simulink model "aa_IOT"  (R2024b)
settings: Solver=VariableStepAuto  StartTime=0.0  StopTime=0.20  RelTol=1e-3
undefined symbols (not defined in the file): Acid, Ion, Lead, Lithium, sigbuilder_block
libraries: spsBreakerLib x120, spsBatteryLib x72, spsSeriesRLCBranchLib x47, spsVoltageMeasurementLib x33, spsIdealSwitchLib x19, spsDiodeLib x10, spsCurrentMeasurementLib x8, spsThyristorLib x6, sldrtlib x4, spsACVoltageSourceLib x3, spsIGBTLib x2, spsPVArrayLib x1
(part 3 of 7)

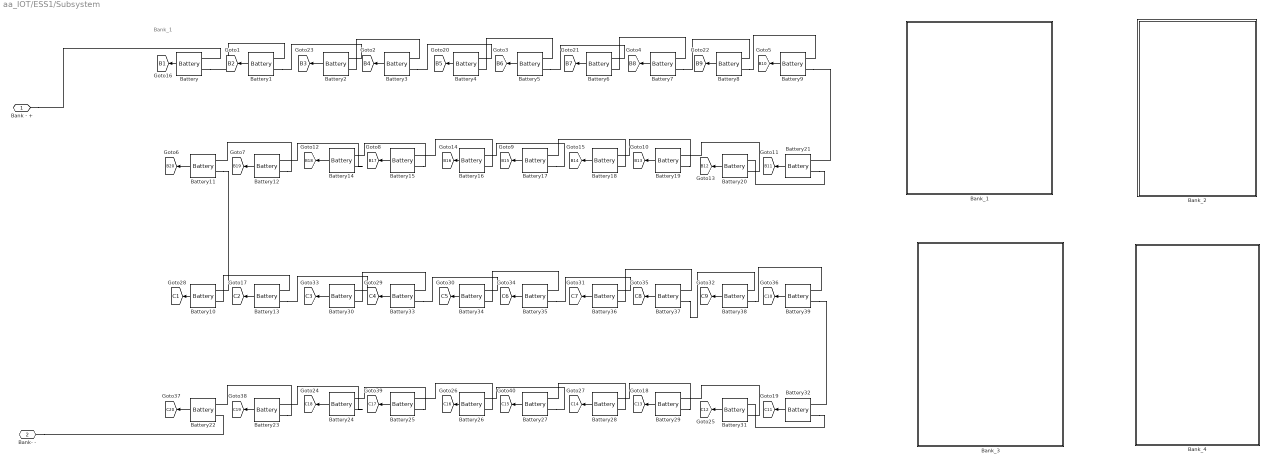
== system aa_IOT/ESS1/Subsystem ==
  note: Bank_1
  Bank_1 : Subsystem
  Bank_2 : Subsystem
  Bank_3 : Subsystem
  Bank_4 : Subsystem
  Battery{,1..39} (40 alike) : spsBatteryLib/Battery  BatType=Lead-Acid  NomV=12  NomQ=100  SOC=80  Batt_Tr=10  PresetModel=on  MaxQ=104.1667  MinV=9  FullV=13.0658  Dis_rate=20  R=0.0012  Normal_OP=31.0278  expZone="[12.2171     0.333333]"
  Bank - + : PMIOPort  Side=Left
  Bank- - : PMIOPort  Port=2  Side=Left
  tag scope: B10=global, B11=global, B12=global, B13=global, B14=global, B15=global, B16=global, B17=global, B18=global, B19=global, B1=global, B20=global, B2=global, B3=global, B4=global, B5=global, B6=global, B7=global, B8=global, B9=global, C10=global, C11=global, C12=global, C13=global, C14=global, C15=global, C16=global, C17=global, C18=global, C19=global, C1=global, C20=global, C2=global, C3=global, C4=global, C5=global, C6=global, C7=global, C8=global, C9=global
  wires:
  Battery1/1 -> [B2]
  Battery5/1 -> [B6]
  Battery25/1 -> [C17]
  Battery20/1 -> [B12]
  Battery34/1 -> [C5]
  Battery28/1 -> [C14]
  Battery4/1 -> [B5]
  Battery16/1 -> [B16]
  Battery2/1 -> [B3]
  Battery18/1 -> [B14]
  Battery14/1 -> [B18]
  Battery8/1 -> [B9]
  Battery6/1 -> [B7]
  Battery17/1 -> [B15]
  Battery24/1 -> [C18]
  Battery9/1 -> [B10]
  Battery12/1 -> [B19]
  Battery15/1 -> [B17]
  Battery21/1 -> [B11]
  Battery11/1 -> [B20]
  Battery10/1 -> [C1]
  Battery19/1 -> [B13]
  Battery3/1 -> [B4]
  Battery7/1 -> [B8]
  Battery27/1 -> [C15]
  Battery13/1 -> [C2]
  Battery/1 -> [B1]
  Battery38/1 -> [C9]
  Battery22/1 -> [C20]
  Battery39/1 -> [C10]
  Battery32/1 -> [C11]
  Battery37/1 -> [C8]
  Battery33/1 -> [C4]
  Battery35/1 -> [C6]
  Battery23/1 -> [C19]
  Battery29/1 -> [C13]
  Battery31/1 -> [C12]
  Battery36/1 -> [C7]
  Battery30/1 -> [C3]
  Battery26/1 -> [C16]
  connections:
  Battery7/LConn2 -- Battery8/LConn1
  Battery20/LConn2 -- Battery19/LConn1
  Battery9/LConn2 -- Battery21/LConn1
  Battery2/LConn2 -- Battery3/LConn1
  Battery13/LConn2 -- Battery30/LConn1
  Battery39/LConn2 -- Battery32/LConn1
  Battery15/LConn2 -- Battery14/LConn1
  Battery16/LConn2 -- Battery15/LConn1
  Battery14/LConn2 -- Battery12/LConn1
  Battery21/LConn2 -- Battery20/LConn1
  Battery6/LConn2 -- Battery7/LConn1
  Battery12/LConn2 -- Battery11/LConn1
  Battery18/LConn2 -- Battery17/LConn1
  Battery17/LConn2 -- Battery16/LConn1
  Battery3/LConn2 -- Battery4/LConn1
  Battery19/LConn2 -- Battery18/LConn1
  Battery8/LConn2 -- Battery9/LConn1
  Battery26/LConn2 -- Battery25/LConn1
  Battery1/LConn2 -- Battery2/LConn1
  Battery4/LConn2 -- Battery5/LConn1
  Battery5/LConn2 -- Battery6/LConn1
  Battery/LConn2 -- Battery1/LConn1
  Battery23/LConn2 -- Battery22/LConn1
  Battery25/LConn2 -- Battery24/LConn1
  Battery10/LConn2 -- Battery13/LConn1
  Battery28/LConn2 -- Battery27/LConn1
  Battery29/LConn2 -- Battery28/LConn1
  Battery33/LConn2 -- Battery34/LConn1
  Battery32/LConn2 -- Battery31/LConn1
  Battery30/LConn2 -- Battery33/LConn1
  Battery34/LConn2 -- Battery35/LConn1
  Battery38/LConn2 -- Battery39/LConn1
  Battery35/LConn2 -- Battery36/LConn1
  Battery24/LConn2 -- Battery23/LConn1
  Battery31/LConn2 -- Battery29/LConn1
  Battery36/LConn2 -- Battery37/LConn1
  Battery37/LConn2 -- Battery38/LConn1
  Battery27/LConn2 -- Battery26/LConn1
  Bank - +/RConn1 -- Battery/LConn1
  Bank- -/RConn1 -- Battery22/LConn2
  Battery11/LConn2 -- Battery10/LConn1

== system aa_IOT/Fast charging controller/Fast charging Switching controller ==
  g1 : Subsystem
  g2 : Subsystem
  g3 : Subsystem
  g4 : Subsystem

== system aa_IOT/Solar/Irradiance  ==
  Demux : Demux  Tag=STV Demux  Outputs=2
      settings: DisplayOption=none
  FromWs : FromWorkspace  Tag=STV FromWs  VariableName=tuvar
      SigBuilderData=|
      | common.afterFinalStr = 'Extrapolate'
      | common.sampleTime = '0'
      | dataSet(1).timeRange = [0 2]
      | dataSet(1).name = 'Constant Irradiance'
      | dataSet(2).timeRange = [0 2]
      | dataSet(2).name = 'Step Irradiance'
      | dataSet(3).timeRange = [0 1]
      | dataSet(3).name = 'Ramp-up/down Irradiance'
      | sbobj.Groups(1).Name = 'Constant Irradiance'
      | sbobj.Groups(1).Signals(1).Name = 'Ir'
      | sbobj.Groups(1).Signals(1).XData = [0 2]
      | sbobj.Groups(1).Signals(1).YData = [1000 1000]
      | sbobj.Groups(1).Signals(2).Name = 'Temp'
      | sbobj.Groups(1).Signals(2).XData = [0 1 1 2]
      | sbobj.Groups(1).Signals(2).YData = [0 0 1 1]
      | sbobj.Groups(1).TimeRange = [0 2]
      | sbobj.Groups(2).Name = 'Step Irradiance'
      | sbobj.Groups(2).Signals(1).Name = 'Ir'
      | sbobj.Groups(2).Signals(1).XData = [0 0.252 0.252 2]
      | sbobj.Groups(2).Signals(1).YData = [600 600 1000 1000]
      | sbobj.Groups(2).Signals(2).Name = 'Temp'
      | sbobj.Groups(2).Signals(2).XData = [0 1 1 2]
      | sbobj.Groups(2).Signals(2).YData = [0 0 1 1]
      | sbobj.Groups(2).TimeRange = [0 2]
      | sbobj.Groups(3).Name = 'Ramp-up/down Irradiance'
      | sbobj.Groups(3).Signals(1).Name = 'Ir'
      | sbobj.Groups(3).Signals(1).XData = [0 0.3 0.3 0.4 0.4 0.5 0.5 1]
      | sbobj.Groups(3).Signals(1).YData = [1000 1000 800 795 600 600 400 395]
      | sbobj.Groups(3).Signals(2).Name = 'Temp'
      | sbobj.Groups(3).Signals(2).XData = [0 1]
      | sbobj.Groups(3).Signals(2).YData = [25 25]
      | sbobj.Groups(3).TimeRange = [0 1]
  Ir : Outport  Tag=STV Outport
  Temp : Outport  Tag=STV Outport  Port=2
  wires:
  Demux/1 -> Ir/1
  FromWs/1 -> Demux/1
  Demux/2 -> Temp/1

== system aa_IOT/Solar/MPPT ==
  "V _ PV " : Inport
  I_PV : Inport  Port=2
  clock : Inport  Port=3
  Embedded MATLAB Function1 : MATLAB Function  TreatAsAtomicUnit=on
  Duty : Outport  VectorParamsAs1DForOutWhenUnconnected=off
  wires:
  Embedded MATLAB Function1/1(D) -> Duty/1
  clock/1 -> Embedded MATLAB Function1/3(T)
  "V _ PV "/1 -> Embedded MATLAB Function1/1(V)
  I_PV/1 -> Embedded MATLAB Function1/2(I)

== system aa_IOT/Solar/Subsystem ==
  Constant : Constant  Value=10000
  Display{1,3..9} (8 alike) : Display
  Mux : Mux  Inputs=8
  Product : Product
  ThingSpeak Output : sldrtlib/Internet of Things/ThingSpeak Output  DrvAddress=2749650  DrvOptions=[1 15 50 66 71 85 71 49 57 55 71 78 77 74 88 48 87 70 97 112 105 46 116 104 105 110 103 115 112 101 97 107 46 99 111 109 0 0 0 0 0 0 0 0 0 0 0 0 0 0 0 0 0 0 0 0 0 0 0 0 0 0 0 0 0 0 0 0 0 0 0 0 0 0 0 0 0 0 0 0 0 0 0 0 0 0 0 0 0 0 0 0 0 0 0 0 0 0 0 0 0 0 0 0 0 0 0 0 0 0 0 0 0 0 0 0 0 0 0 0 0 0 0 0 0 0 0 0 0 0 0 0 0 0 0 0 0 0 0 0 0 0 0 0 0 0 0 0 0 0 0 0 0 0 0 0 0 0 0 0 0 0 0 0 0 0 0 0 0 0 0 0 0 0 0 0 0 0 0 0 0 0 0 0 0 0 0 0 0 0 0 0 0 0 0 0 0 0 0 0 0 0 0 0 0 0 0 0 0 0 0 0 0 0 0 0 0 0 0 0 0 0 0 0 0 0 0 0 0 0 0 0 0 0 0 0 0 0 0 0 0 0 0 0 0 0 0 0 0 0 0 0 0 0 0 0]  SampleTime=0.1  MaxMissedTicks=10000000000000000000000000000000000000000000  ShowMissedTicks=off  YieldWhenWaiting=off  ChannelFields=[1 2 3 4 5 6 7 8]  OptParam=0  InitialValue=[]  FinalValue=[]
  wires:
  [solar_v] -> Mux/1, Display9/1
  [solar_i] -> Mux/2, Display3/1
  [solar_out_p] -> Mux/8, Display7/1
  [solar_irr] -> Mux/5, Display4/1
  [solar_out_i] -> Mux/7, Display8/1
  [solar_out_v] -> Mux/6, Display6/1
  [solar_temp] -> Mux/4, Display5/1
  Mux/1 -> ThingSpeak Output/1
  Product/1 -> Mux/3, Display1/1
  [solar_p] -> Product/2
  Constant/1 -> Product/1

== system aa_IOT/Subsystem/Car Charging Calculator ==
  note: Car Charging Calculator
  note: Car Batttery KWh
  note: Volatge
  note: Current
  note: Time Required in hr
  note: Power in Kw
  note: Power Valiabililty
  Car Battery KWh : Constant  Value=600
  Current : Constant  Value=20
  Display : CustomWebBlock  LabelPosition=Hide  ShowInitialText=on  Configuration="{\"components\":[{\"name\":\"DisplayComponent\",\"settings\":{\"bold\":false,\"font\":\"DSEG7 Classic\",\"fontColor\":[255,255,200],\"fontSize\":\"14\",\"format\":\"short\",\"formatString\":\"%d\",\"italic\":false,\"position\":[0,0,1,1],\"underline\":false}},{\"name\":\"BackgroundImageComponent\",\"settings\":{\"image\":{\"size\":[300,80],\"src\":\"data:image\\/svg+xml;base64,PHN2ZyBpZD0iZnJhbWUiIHhtbG5zPSJodHRwOi8vd3d3LnczLm9yZy8yMDAwL3N2ZyIgeG1sbnM6eGxpbms9Imh0dHA6Ly93d3cudzMub3JnLzE5OTkveGxpbmsiIHZpZXdCb3g9IjAgMCAzODAgMTAxIj48ZGVmcz48c3R5bGU+LmNscy0xe2ZpbGw6IzAwMmI0Mjt9LmNscy0ye2ZpbGw6IzQyNzA4Mjt9LmNscy0ze2ZpbGw6dXJsKCNyYWRpYWwtZ3JhZGllbnQpO308L3N0eWxlPjxyYWRpYWxHcmFkaWVudCBpZD0icmFkaWFsLWdyYWRpZW50IiBjeD0iMTkwIiBjeT0iNTAuNSIgcj0iMjY5LjIxIiBncmFkaWVudFVuaXRzPSJ1c2VyU3BhY2VPblVzZSI+PHN0b3Agb2Zmc2V0PSIwLjAxIiBzdG9wLWNvbG9yPSIjM2U0ZjU4Ii8+PHN0b3Agb2Zmc2V0PSIwLjA2IiBzdG9wLWNvbG9yPSIjNDQ1NzYxIi8+PHN0b3Agb2Zmc2V0PSIwLjE1IiBzdG9wLWNvbG9yPSIjNTU2YTc2Ii8+PHN0b3Agb2Zmc2V0PSIwLjI1IiBzdG9wLWNvbG9yPSIjNmQ4ODk1Ii8+PHN0b3Agb2Zmc2V0PSIwLjM4IiBzdG9wLWNvbG9yPSIjOGZiMmMzIi8+PHN0b3Agb2Zmc2V0PSIwLjUyIiBzdG9wLWNvbG9yPSIjYjZlNGZhIi8+PHN0b3Agb2Zmc2V0PSIxIiBzdG9wLWNvbG9yPSIjMTU0NjU3Ii8+PC9yYWRpYWxHcmFkaWVudD48L2RlZnM+PGcgaWQ9IkxheWVyXzIiIGRhdGEtbmFtZT0iTGF5ZXIgMiI+PGcgaWQ9IkxheWVyXzEtMiIgZGF0YS1uYW1lPSJMYXllciAxLTIiPjxyZWN0IGlkPSJyZWN0MTAzNiIgY2xhc3M9ImNscy0xIiB4PSIxMSIgeT0iMTEiIHdpZHRoPSIzNTgiIGhlaWdodD0iNzkiLz48cGF0aCBpZD0icGF0aDEwMzgiIGNsYXNzPSJjbHMtMiIgZD0iTTgsOFY5M0gzNzJWOFpNMzY5LDkwSDExVjExSDM2OVoiLz48cGF0aCBpZD0icGF0aDEwNDAiIGNsYXNzPSJjbHMtMyIgZD0iTTAsMFYxMDFIMzgwVjBaTTM3Miw5M0g4VjhIMzcyWiIvPjwvZz48L2c+PC9zdmc+\",\"srcOrientation\":\"Right\"},\"position\":[0,0,1,1],\"scaleMode\":\"0\"}},{\"name\":\"ForegroundImageComponent\",\"settings\":{\"angle\":0,\"image\":{\"size\":[0,0],\"src\":\"default\"},\"isForeground\":1,\"position\":[0,0,1,1],\"scaleMode\":\"0\"}}],\"settings\":{\"BindingType\":\"signal\",\"aspectRatio\":1.032258064516129,\"backgroundColor\":[0,0,0,\"1\"],\"backgroundOffset\":0.14,\"backgroundOpacity\":1,\"fixedAspectRatio\":\"on\",\"showBackgroundColor\":false,\"value\":0,\"version\":\"R2023b\"},\"type\":\"Display\"}"
  Display1 : CustomWebBlock  LabelPosition=Hide  ShowInitialText=on  Configuration="{\"components\":[{\"name\":\"DisplayComponent\",\"settings\":{\"bold\":false,\"font\":\"DSEG7 Classic\",\"fontColor\":[255,255,200],\"fontSize\":\"14\",\"format\":\"short\",\"formatString\":\"%d\",\"italic\":false,\"position\":[0,0,1,1],\"underline\":false}},{\"name\":\"BackgroundImageComponent\",\"settings\":{\"image\":{\"size\":[300,80],\"src\":\"data:image\\/svg+xml;base64,PHN2ZyBpZD0iZnJhbWUiIHhtbG5zPSJodHRwOi8vd3d3LnczLm9yZy8yMDAwL3N2ZyIgeG1sbnM6eGxpbms9Imh0dHA6Ly93d3cudzMub3JnLzE5OTkveGxpbmsiIHZpZXdCb3g9IjAgMCAzODAgMTAxIj48ZGVmcz48c3R5bGU+LmNscy0xe2ZpbGw6IzAwMmI0Mjt9LmNscy0ye2ZpbGw6IzQyNzA4Mjt9LmNscy0ze2ZpbGw6dXJsKCNyYWRpYWwtZ3JhZGllbnQpO308L3N0eWxlPjxyYWRpYWxHcmFkaWVudCBpZD0icmFkaWFsLWdyYWRpZW50IiBjeD0iMTkwIiBjeT0iNTAuNSIgcj0iMjY5LjIxIiBncmFkaWVudFVuaXRzPSJ1c2VyU3BhY2VPblVzZSI+PHN0b3Agb2Zmc2V0PSIwLjAxIiBzdG9wLWNvbG9yPSIjM2U0ZjU4Ii8+PHN0b3Agb2Zmc2V0PSIwLjA2IiBzdG9wLWNvbG9yPSIjNDQ1NzYxIi8+PHN0b3Agb2Zmc2V0PSIwLjE1IiBzdG9wLWNvbG9yPSIjNTU2YTc2Ii8+PHN0b3Agb2Zmc2V0PSIwLjI1IiBzdG9wLWNvbG9yPSIjNmQ4ODk1Ii8+PHN0b3Agb2Zmc2V0PSIwLjM4IiBzdG9wLWNvbG9yPSIjOGZiMmMzIi8+PHN0b3Agb2Zmc2V0PSIwLjUyIiBzdG9wLWNvbG9yPSIjYjZlNGZhIi8+PHN0b3Agb2Zmc2V0PSIxIiBzdG9wLWNvbG9yPSIjMTU0NjU3Ii8+PC9yYWRpYWxHcmFkaWVudD48L2RlZnM+PGcgaWQ9IkxheWVyXzIiIGRhdGEtbmFtZT0iTGF5ZXIgMiI+PGcgaWQ9IkxheWVyXzEtMiIgZGF0YS1uYW1lPSJMYXllciAxLTIiPjxyZWN0IGlkPSJyZWN0MTAzNiIgY2xhc3M9ImNscy0xIiB4PSIxMSIgeT0iMTEiIHdpZHRoPSIzNTgiIGhlaWdodD0iNzkiLz48cGF0aCBpZD0icGF0aDEwMzgiIGNsYXNzPSJjbHMtMiIgZD0iTTgsOFY5M0gzNzJWOFpNMzY5LDkwSDExVjExSDM2OVoiLz48cGF0aCBpZD0icGF0aDEwNDAiIGNsYXNzPSJjbHMtMyIgZD0iTTAsMFYxMDFIMzgwVjBaTTM3Miw5M0g4VjhIMzcyWiIvPjwvZz48L2c+PC9zdmc+\",\"srcOrientation\":\"Right\"},\"position\":[0,0,1,1],\"scaleMode\":\"0\"}},{\"name\":\"ForegroundImageComponent\",\"settings\":{\"angle\":0,\"image\":{\"size\":[0,0],\"src\":\"default\"},\"isForeground\":1,\"position\":[0,0,1,1],\"scaleMode\":\"0\"}}],\"settings\":{\"BindingType\":\"signal\",\"aspectRatio\":1.032258064516129,\"backgroundColor\":[0,0,0,\"1\"],\"backgroundOffset\":0.14,\"backgroundOpacity\":1,\"fixedAspectRatio\":\"on\",\"showBackgroundColor\":false,\"value\":0,\"version\":\"R2023b\"},\"type\":\"Display\"}"
  Display2 : CustomWebBlock  LabelPosition=Hide  ShowInitialText=on  Configuration="{\"components\":[{\"name\":\"DisplayComponent\",\"settings\":{\"bold\":false,\"font\":\"DSEG7 Classic\",\"fontColor\":[255,255,200],\"fontSize\":\"14\",\"format\":\"short\",\"formatString\":\"%d\",\"italic\":false,\"position\":[0,0,1,1],\"underline\":false}},{\"name\":\"BackgroundImageComponent\",\"settings\":{\"image\":{\"size\":[300,80],\"src\":\"data:image\\/svg+xml;base64,PHN2ZyBpZD0iZnJhbWUiIHhtbG5zPSJodHRwOi8vd3d3LnczLm9yZy8yMDAwL3N2ZyIgeG1sbnM6eGxpbms9Imh0dHA6Ly93d3cudzMub3JnLzE5OTkveGxpbmsiIHZpZXdCb3g9IjAgMCAzODAgMTAxIj48ZGVmcz48c3R5bGU+LmNscy0xe2ZpbGw6IzAwMmI0Mjt9LmNscy0ye2ZpbGw6IzQyNzA4Mjt9LmNscy0ze2ZpbGw6dXJsKCNyYWRpYWwtZ3JhZGllbnQpO308L3N0eWxlPjxyYWRpYWxHcmFkaWVudCBpZD0icmFkaWFsLWdyYWRpZW50IiBjeD0iMTkwIiBjeT0iNTAuNSIgcj0iMjY5LjIxIiBncmFkaWVudFVuaXRzPSJ1c2VyU3BhY2VPblVzZSI+PHN0b3Agb2Zmc2V0PSIwLjAxIiBzdG9wLWNvbG9yPSIjM2U0ZjU4Ii8+PHN0b3Agb2Zmc2V0PSIwLjA2IiBzdG9wLWNvbG9yPSIjNDQ1NzYxIi8+PHN0b3Agb2Zmc2V0PSIwLjE1IiBzdG9wLWNvbG9yPSIjNTU2YTc2Ii8+PHN0b3Agb2Zmc2V0PSIwLjI1IiBzdG9wLWNvbG9yPSIjNmQ4ODk1Ii8+PHN0b3Agb2Zmc2V0PSIwLjM4IiBzdG9wLWNvbG9yPSIjOGZiMmMzIi8+PHN0b3Agb2Zmc2V0PSIwLjUyIiBzdG9wLWNvbG9yPSIjYjZlNGZhIi8+PHN0b3Agb2Zmc2V0PSIxIiBzdG9wLWNvbG9yPSIjMTU0NjU3Ii8+PC9yYWRpYWxHcmFkaWVudD48L2RlZnM+PGcgaWQ9IkxheWVyXzIiIGRhdGEtbmFtZT0iTGF5ZXIgMiI+PGcgaWQ9IkxheWVyXzEtMiIgZGF0YS1uYW1lPSJMYXllciAxLTIiPjxyZWN0IGlkPSJyZWN0MTAzNiIgY2xhc3M9ImNscy0xIiB4PSIxMSIgeT0iMTEiIHdpZHRoPSIzNTgiIGhlaWdodD0iNzkiLz48cGF0aCBpZD0icGF0aDEwMzgiIGNsYXNzPSJjbHMtMiIgZD0iTTgsOFY5M0gzNzJWOFpNMzY5LDkwSDExVjExSDM2OVoiLz48cGF0aCBpZD0icGF0aDEwNDAiIGNsYXNzPSJjbHMtMyIgZD0iTTAsMFYxMDFIMzgwVjBaTTM3Miw5M0g4VjhIMzcyWiIvPjwvZz48L2c+PC9zdmc+\",\"srcOrientation\":\"Right\"},\"position\":[0,0,1,1],\"scaleMode\":\"0\"}},{\"name\":\"ForegroundImageComponent\",\"settings\":{\"angle\":0,\"image\":{\"size\":[0,0],\"src\":\"default\"},\"isForeground\":1,\"position\":[0,0,1,1],\"scaleMode\":\"0\"}}],\"settings\":{\"BindingType\":\"signal\",\"aspectRatio\":1.032258064516129,\"backgroundColor\":[0,0,0,\"1\"],\"backgroundOffset\":0.14,\"backgroundOpacity\":1,\"fixedAspectRatio\":\"on\",\"showBackgroundColor\":false,\"value\":0,\"version\":\"R2023b\"},\"type\":\"Display\"}"
  Display3 : CustomWebBlock  LabelPosition=Hide  ShowInitialText=on  Configuration="{\"components\":[{\"name\":\"DisplayComponent\",\"settings\":{\"bold\":false,\"font\":\"DSEG7 Classic\",\"fontColor\":[255,255,200],\"fontSize\":\"14\",\"format\":\"shortG\",\"formatString\":\"%d\",\"italic\":false,\"position\":[0,0,1,1],\"underline\":false}},{\"name\":\"BackgroundImageComponent\",\"settings\":{\"image\":{\"size\":[300,80],\"src\":\"data:image\\/svg+xml;base64,PHN2ZyBpZD0iZnJhbWUiIHhtbG5zPSJodHRwOi8vd3d3LnczLm9yZy8yMDAwL3N2ZyIgeG1sbnM6eGxpbms9Imh0dHA6Ly93d3cudzMub3JnLzE5OTkveGxpbmsiIHZpZXdCb3g9IjAgMCAzODAgMTAxIj48ZGVmcz48c3R5bGU+LmNscy0xe2ZpbGw6IzAwMmI0Mjt9LmNscy0ye2ZpbGw6IzQyNzA4Mjt9LmNscy0ze2ZpbGw6dXJsKCNyYWRpYWwtZ3JhZGllbnQpO308L3N0eWxlPjxyYWRpYWxHcmFkaWVudCBpZD0icmFkaWFsLWdyYWRpZW50IiBjeD0iMTkwIiBjeT0iNTAuNSIgcj0iMjY5LjIxIiBncmFkaWVudFVuaXRzPSJ1c2VyU3BhY2VPblVzZSI+PHN0b3Agb2Zmc2V0PSIwLjAxIiBzdG9wLWNvbG9yPSIjM2U0ZjU4Ii8+PHN0b3Agb2Zmc2V0PSIwLjA2IiBzdG9wLWNvbG9yPSIjNDQ1NzYxIi8+PHN0b3Agb2Zmc2V0PSIwLjE1IiBzdG9wLWNvbG9yPSIjNTU2YTc2Ii8+PHN0b3Agb2Zmc2V0PSIwLjI1IiBzdG9wLWNvbG9yPSIjNmQ4ODk1Ii8+PHN0b3Agb2Zmc2V0PSIwLjM4IiBzdG9wLWNvbG9yPSIjOGZiMmMzIi8+PHN0b3Agb2Zmc2V0PSIwLjUyIiBzdG9wLWNvbG9yPSIjYjZlNGZhIi8+PHN0b3Agb2Zmc2V0PSIxIiBzdG9wLWNvbG9yPSIjMTU0NjU3Ii8+PC9yYWRpYWxHcmFkaWVudD48L2RlZnM+PGcgaWQ9IkxheWVyXzIiIGRhdGEtbmFtZT0iTGF5ZXIgMiI+PGcgaWQ9IkxheWVyXzEtMiIgZGF0YS1uYW1lPSJMYXllciAxLTIiPjxyZWN0IGlkPSJyZWN0MTAzNiIgY2xhc3M9ImNscy0xIiB4PSIxMSIgeT0iMTEiIHdpZHRoPSIzNTgiIGhlaWdodD0iNzkiLz48cGF0aCBpZD0icGF0aDEwMzgiIGNsYXNzPSJjbHMtMiIgZD0iTTgsOFY5M0gzNzJWOFpNMzY5LDkwSDExVjExSDM2OVoiLz48cGF0aCBpZD0icGF0aDEwNDAiIGNsYXNzPSJjbHMtMyIgZD0iTTAsMFYxMDFIMzgwVjBaTTM3Miw5M0g4VjhIMzcyWiIvPjwvZz48L2c+PC9zdmc+\",\"srcOrientation\":\"Right\"},\"position\":[0,0,1,1],\"scaleMode\":\"0\"}},{\"name\":\"ForegroundImageComponent\",\"settings\":{\"angle\":0,\"image\":{\"size\":[0,0],\"src\":\"default\"},\"isForeground\":1,\"position\":[0,0,1,1],\"scaleMode\":\"0\"}}],\"settings\":{\"BindingType\":\"signal\",\"aspectRatio\":1.032258064516129,\"backgroundColor\":[0,0,0,\"1\"],\"backgroundOffset\":0.14,\"backgroundOpacity\":1,\"fixedAspectRatio\":\"on\",\"showBackgroundColor\":false,\"value\":0,\"version\":\"R2023b\"},\"type\":\"Display\"}"
  Display4 : CustomWebBlock  LabelPosition=Hide  ShowInitialText=on  Configuration="{\"components\":[{\"name\":\"DisplayComponent\",\"settings\":{\"bold\":false,\"font\":\"DSEG7 Classic\",\"fontColor\":[255,255,200],\"fontSize\":\"14\",\"format\":\"shortG\",\"formatString\":\"%d\",\"italic\":false,\"position\":[0,0,1,1],\"underline\":false}},{\"name\":\"BackgroundImageComponent\",\"settings\":{\"image\":{\"size\":[300,80],\"src\":\"data:image\\/svg+xml;base64,PHN2ZyBpZD0iZnJhbWUiIHhtbG5zPSJodHRwOi8vd3d3LnczLm9yZy8yMDAwL3N2ZyIgeG1sbnM6eGxpbms9Imh0dHA6Ly93d3cudzMub3JnLzE5OTkveGxpbmsiIHZpZXdCb3g9IjAgMCAzODAgMTAxIj48ZGVmcz48c3R5bGU+LmNscy0xe2ZpbGw6IzAwMmI0Mjt9LmNscy0ye2ZpbGw6IzQyNzA4Mjt9LmNscy0ze2ZpbGw6dXJsKCNyYWRpYWwtZ3JhZGllbnQpO308L3N0eWxlPjxyYWRpYWxHcmFkaWVudCBpZD0icmFkaWFsLWdyYWRpZW50IiBjeD0iMTkwIiBjeT0iNTAuNSIgcj0iMjY5LjIxIiBncmFkaWVudFVuaXRzPSJ1c2VyU3BhY2VPblVzZSI+PHN0b3Agb2Zmc2V0PSIwLjAxIiBzdG9wLWNvbG9yPSIjM2U0ZjU4Ii8+PHN0b3Agb2Zmc2V0PSIwLjA2IiBzdG9wLWNvbG9yPSIjNDQ1NzYxIi8+PHN0b3Agb2Zmc2V0PSIwLjE1IiBzdG9wLWNvbG9yPSIjNTU2YTc2Ii8+PHN0b3Agb2Zmc2V0PSIwLjI1IiBzdG9wLWNvbG9yPSIjNmQ4ODk1Ii8+PHN0b3Agb2Zmc2V0PSIwLjM4IiBzdG9wLWNvbG9yPSIjOGZiMmMzIi8+PHN0b3Agb2Zmc2V0PSIwLjUyIiBzdG9wLWNvbG9yPSIjYjZlNGZhIi8+PHN0b3Agb2Zmc2V0PSIxIiBzdG9wLWNvbG9yPSIjMTU0NjU3Ii8+PC9yYWRpYWxHcmFkaWVudD48L2RlZnM+PGcgaWQ9IkxheWVyXzIiIGRhdGEtbmFtZT0iTGF5ZXIgMiI+PGcgaWQ9IkxheWVyXzEtMiIgZGF0YS1uYW1lPSJMYXllciAxLTIiPjxyZWN0IGlkPSJyZWN0MTAzNiIgY2xhc3M9ImNscy0xIiB4PSIxMSIgeT0iMTEiIHdpZHRoPSIzNTgiIGhlaWdodD0iNzkiLz48cGF0aCBpZD0icGF0aDEwMzgiIGNsYXNzPSJjbHMtMiIgZD0iTTgsOFY5M0gzNzJWOFpNMzY5LDkwSDExVjExSDM2OVoiLz48cGF0aCBpZD0icGF0aDEwNDAiIGNsYXNzPSJjbHMtMyIgZD0iTTAsMFYxMDFIMzgwVjBaTTM3Miw5M0g4VjhIMzcyWiIvPjwvZz48L2c+PC9zdmc+\",\"srcOrientation\":\"Right\"},\"position\":[0,0,1,1],\"scaleMode\":\"0\"}},{\"name\":\"ForegroundImageComponent\",\"settings\":{\"angle\":0,\"image\":{\"size\":[0,0],\"src\":\"default\"},\"isForeground\":1,\"position\":[0,0,1,1],\"scaleMode\":\"0\"}}],\"settings\":{\"BindingType\":\"signal\",\"aspectRatio\":1.032258064516129,\"backgroundColor\":[0,0,0,\"1\"],\"backgroundOffset\":0.14,\"backgroundOpacity\":1,\"fixedAspectRatio\":\"on\",\"showBackgroundColor\":false,\"value\":0,\"version\":\"R2023b\"},\"type\":\"Display\"}"
  Lamp : LampBlock  Icon=Check2
  Power : Display
  Subsystem9 : Subsystem
  Time : Display
  Voltage : Constant  Value=240
  wires:
  Voltage/1 -> Subsystem9/2(In2)
  Current/1 -> Subsystem9/3(In3)
  Subsystem9/1(Out1) -> Time/1
  Car Battery KWh/1 -> Subsystem9/1(In1)
  Subsystem9/2(Out2) -> Power/1

== system aa_IOT/Subsystem11/. ==
  Battery : spsBatteryLib/Battery  BatType=Lithium-Ion  NomV=12  NomQ=10  SOC=95  Batt_Tr=30  PresetModel=on  MaxQ=10  MinV=9  FullV=13.9678  Dis_rate=4.3478  R=0.012  Normal_OP=9.0435  expZone="[12.9646     0.491304]"
  Breaker{,1..3} (4 alike) : spsBreakerLib/Breaker  InitialState=0  SwitchingTimes="[1/60  5/60]"  External=on  BreakerResistance=0.01  SnubberResistance=1e6  SnubberCapacitance=inf  Measurements=None  MoreParameters=on  NoBreakLoop=off
  Bus Selector : BusSelector  OutputSignals=SOC (%),Current (A),Voltage (V)
  Constant : Constant  Value=1000000
  Constant1 : Constant  Value=30
  Product : Product
  Scope : Scope  NumInputPorts=3
  Series RLC Branch : spsSeriesRLCBranchLib/Series RLC Branch  LConnTagsString=__new0  RConnTagsString=__new0  BranchType=R  Resistance=1  Inductance=1e-3  SetiL0=off  InitialCurrent=0  Capacitance=1e-6  Setx0=off  InitialVoltage=0  Measurements=None
  + : PMIOPort  Side=Right
  - : PMIOPort  Port=2  Side=Right
  tag scope: batt_ava=global, batt_power=global, batt_soc=global, batt_voltage=global, s1=global
  wires:
  Battery/1 -> Bus Selector/1
  [c1] -> Breaker3/1, Breaker/1
  [d1] -> Breaker1/1, Breaker2/1
  Bus Selector/3 -> [batt_voltage], Scope/3  "<Voltage (V)>"
  Bus Selector/1 -> [s1], [batt_soc], Scope/1  "<SOC (%)>"
  Bus Selector/2 -> Product/1  "<Current (A)>"
  Constant/1 -> Product/2
  Product/1 -> [batt_power], Scope/2
  Constant1/1 -> [batt_ava]
  connections:
  Breaker2/LConn1 -- Breaker3/RConn1 -- Battery/LConn2
  Breaker1/LConn1 -- Battery/LConn1 -- Breaker/RConn1
  +/RConn1 -- Breaker/LConn1
  Series RLC Branch/LConn1 -- Breaker2/RConn1
  Series RLC Branch/RConn1 -- Breaker1/RConn1
  -/RConn1 -- Breaker3/LConn1

== system aa_IOT/Subsystem11/DC - DC Converter ==
  C : spsSeriesRLCBranchLib/Series RLC Branch  LConnTagsString=__new0  RConnTagsString=__new0  BranchType=C  Resistance=0.01  Inductance=1e-3  SetiL0=off  InitialCurrent=0  Capacitance=1000e-6  Setx0=on  InitialVoltage=200  Measurements=None
  Diode : spsDiodeLib/Diode  Ron=0.001  Lon=0  Vf=1.1  IC=0  UseSnubber=off  Rs=500  Cs=250e-9  Measurements=off
  Diode2 : spsDiodeLib/Diode  Ron=0.001  Lon=0  Vf=0.7  IC=0  UseSnubber=off  Rs=500  Cs=250e-9  Measurements=off
  Display1 : Display
  Display2 : Display
  IGBT : spsIGBTLib/IGBT  Ron=0.001  Lon=0  Vf=1.1  Tf=1e-6  Tt=2e-6  IC=0  Rs=1e5  Cs=inf  Measurements=off
  Pulse Generator : DiscretePulseGenerator  PulseType=Time based  Period=10  PulseWidth=5
  RL : spsSeriesRLCBranchLib/Series RLC Branch  LConnTagsString=__new0  RConnTagsString=__new0  BranchType=RL  Resistance=0.05  Inductance=470e-6  SetiL0=off  InitialCurrent=0  Capacitance=1e-6  Setx0=off  InitialVoltage=0  Measurements=None
  Voltage Measurement1 : spsVoltageMeasurementLib/Voltage Measurement  PhasorSimulation=off  OutputType=Complex  PSBequivalent=0
  Voltage Measurement2 : spsVoltageMeasurementLib/Voltage Measurement  PhasorSimulation=off  OutputType=Complex  PSBequivalent=0
  DC + : PMIOPort  Side=Right
  solar panel + : PMIOPort  Port=2  Side=Left
  solar panel - : PMIOPort  Port=3  Side=Left
  DC - : PMIOPort  Port=4  Side=Right
  wires:
  Pulse Generator/1 -> IGBT/1
  Voltage Measurement1/1 -> Display1/1
  Voltage Measurement2/1 -> Display2/1
  connections:
  DC +/RConn1 -- Diode/RConn1 -- Voltage Measurement2/LConn1
  Diode2/RConn1 -- C/LConn1 -- RL/LConn1
  Diode/LConn1 -- RL/RConn1 -- IGBT/LConn1
  Diode2/LConn1 -- solar panel +/RConn1 -- Voltage Measurement1/LConn1
  DC -/RConn1 -- C/RConn1 -- Voltage Measurement1/LConn2 -- solar panel -/RConn1 -- IGBT/RConn1 -- Voltage Measurement2/LConn2

== system aa_IOT/Subsystem11/Subsystem ==
  Battery : spsBatteryLib/Battery  BatType=Lithium-Ion  NomV=12  NomQ=10  SOC=95  Batt_Tr=30  PresetModel=on  MaxQ=10  MinV=9  FullV=13.9678  Dis_rate=4.3478  R=0.012  Normal_OP=9.0435  expZone="[12.9646     0.491304]"
  Breaker{,1..3} (4 alike) : spsBreakerLib/Breaker  InitialState=0  SwitchingTimes="[1/60  5/60]"  External=on  BreakerResistance=0.01  SnubberResistance=1e6  SnubberCapacitance=inf  Measurements=None  MoreParameters=on  NoBreakLoop=off
  Bus Selector : BusSelector  OutputSignals=SOC (%),Current (A),Voltage (V)
  Scope : Scope  NumInputPorts=3
  Series RLC Branch : spsSeriesRLCBranchLib/Series RLC Branch  LConnTagsString=__new0  RConnTagsString=__new0  BranchType=R  Resistance=1  Inductance=1e-3  SetiL0=off  InitialCurrent=0  Capacitance=1e-6  Setx0=off  InitialVoltage=0  Measurements=None
  + : PMIOPort  Side=Right
  - : PMIOPort  Port=2  Side=Right
  tag scope: s5=global
  wires:
  Battery/1 -> Bus Selector/1
  [c5] -> Breaker3/1, Breaker/1
  Bus Selector/2 -> Scope/2  "<Current (A)>"
  [d5] -> Breaker1/1, Breaker2/1
  Bus Selector/3 -> Scope/3  "<Voltage (V)>"
  Bus Selector/1 -> [s5], Scope/1  "<SOC (%)>"
  connections:
  Breaker2/LConn1 -- Breaker3/RConn1 -- Battery/LConn2
  Breaker1/LConn1 -- Battery/LConn1 -- Breaker/RConn1
  +/RConn1 -- Breaker/LConn1
  Series RLC Branch/LConn1 -- Breaker2/RConn1
  Series RLC Branch/RConn1 -- Breaker1/RConn1
  -/RConn1 -- Breaker3/LConn1

== system aa_IOT/Subsystem11/Subsystem10 ==
  Battery : spsBatteryLib/Battery  BatType=Lithium-Ion  NomV=12  NomQ=10  SOC=95  Batt_Tr=30  PresetModel=on  MaxQ=10  MinV=9  FullV=13.9678  Dis_rate=4.3478  R=0.012  Normal_OP=9.0435  expZone="[12.9646     0.491304]"
  Breaker{,1..3} (4 alike) : spsBreakerLib/Breaker  InitialState=0  SwitchingTimes="[1/60  5/60]"  External=on  BreakerResistance=0.01  SnubberResistance=1e6  SnubberCapacitance=inf  Measurements=None  MoreParameters=on  NoBreakLoop=off
  Bus Selector : BusSelector  OutputSignals=SOC (%),Current (A),Voltage (V)
  Display : Display
  MATLAB Function : MATLAB Function  TreatAsAtomicUnit=on
  Scope : Scope  NumInputPorts=3
  Series RLC Branch : spsSeriesRLCBranchLib/Series RLC Branch  LConnTagsString=__new0  RConnTagsString=__new0  BranchType=R  Resistance=1  Inductance=1e-3  SetiL0=off  InitialCurrent=0  Capacitance=1e-6  Setx0=off  InitialVoltage=0  Measurements=None
  + : PMIOPort  Side=Right
  - : PMIOPort  Port=2  Side=Right
  tag scope: s16=global
  wires:
  Battery/1 -> Bus Selector/1
  [c16] -> Breaker3/1, Breaker/1
  Bus Selector/2 -> MATLAB Function/3(Current), Scope/2  "<Current (A)>"
  [d16] -> Breaker1/1, Breaker2/1
  Bus Selector/3 -> MATLAB Function/2(Voltage), Scope/3  "<Voltage (V)>"
  Bus Selector/1 -> [s16], MATLAB Function/1(SOC), Scope/1  "<SOC (%)>"
  MATLAB Function/1(output) -> Display/1
  connections:
  Breaker2/LConn1 -- Breaker3/RConn1 -- Battery/LConn2
  Breaker1/LConn1 -- Battery/LConn1 -- Breaker/RConn1
  +/RConn1 -- Breaker/LConn1
  Series RLC Branch/LConn1 -- Breaker2/RConn1
  Series RLC Branch/RConn1 -- Breaker1/RConn1
  -/RConn1 -- Breaker3/LConn1

== system aa_IOT/Subsystem11/Subsystem11 ==
  Battery : spsBatteryLib/Battery  BatType=Lithium-Ion  NomV=12  NomQ=10  SOC=95  Batt_Tr=30  PresetModel=on  MaxQ=10  MinV=9  FullV=13.9678  Dis_rate=4.3478  R=0.012  Normal_OP=9.0435  expZone="[12.9646     0.491304]"
  Breaker{,1..3} (4 alike) : spsBreakerLib/Breaker  InitialState=0  SwitchingTimes="[1/60  5/60]"  External=on  BreakerResistance=0.01  SnubberResistance=1e6  SnubberCapacitance=inf  Measurements=None  MoreParameters=on  NoBreakLoop=off
  Bus Selector : BusSelector  OutputSignals=SOC (%),Current (A),Voltage (V)
  Display : Display
  MATLAB Function : MATLAB Function  TreatAsAtomicUnit=on
  Scope : Scope  NumInputPorts=3
  Series RLC Branch : spsSeriesRLCBranchLib/Series RLC Branch  LConnTagsString=__new0  RConnTagsString=__new0  BranchType=R  Resistance=1  Inductance=1e-3  SetiL0=off  InitialCurrent=0  Capacitance=1e-6  Setx0=off  InitialVoltage=0  Measurements=None
  + : PMIOPort  Side=Right
  - : PMIOPort  Port=2  Side=Right
  tag scope: s18=global
  wires:
  Battery/1 -> Bus Selector/1
  [c18] -> Breaker3/1, Breaker/1
  Bus Selector/2 -> MATLAB Function/3(Current), Scope/2  "<Current (A)>"
  [d18] -> Breaker1/1, Breaker2/1
  Bus Selector/3 -> MATLAB Function/2(Voltage), Scope/3  "<Voltage (V)>"
  Bus Selector/1 -> [s18], MATLAB Function/1(SOC), Scope/1  "<SOC (%)>"
  MATLAB Function/1(output) -> Display/1
  connections:
  Breaker2/LConn1 -- Breaker3/RConn1 -- Battery/LConn2
  Breaker1/LConn1 -- Battery/LConn1 -- Breaker/RConn1
  +/RConn1 -- Breaker/LConn1
  Series RLC Branch/LConn1 -- Breaker2/RConn1
  Series RLC Branch/RConn1 -- Breaker1/RConn1
  -/RConn1 -- Breaker3/LConn1

== system aa_IOT/Subsystem11/Subsystem12 ==
  Battery : spsBatteryLib/Battery  BatType=Lithium-Ion  NomV=12  NomQ=10  SOC=95  Batt_Tr=30  PresetModel=on  MaxQ=10  MinV=9  FullV=13.9678  Dis_rate=4.3478  R=0.012  Normal_OP=9.0435  expZone="[12.9646     0.491304]"
  Breaker{,1..3} (4 alike) : spsBreakerLib/Breaker  InitialState=0  SwitchingTimes="[1/60  5/60]"  External=on  BreakerResistance=0.01  SnubberResistance=1e6  SnubberCapacitance=inf  Measurements=None  MoreParameters=on  NoBreakLoop=off
  Bus Selector : BusSelector  OutputSignals=SOC (%),Current (A),Voltage (V)
  Scope : Scope  NumInputPorts=3
  Series RLC Branch : spsSeriesRLCBranchLib/Series RLC Branch  LConnTagsString=__new0  RConnTagsString=__new0  BranchType=R  Resistance=1  Inductance=1e-3  SetiL0=off  InitialCurrent=0  Capacitance=1e-6  Setx0=off  InitialVoltage=0  Measurements=None
  + : PMIOPort  Side=Right
  - : PMIOPort  Port=2  Side=Right
  tag scope: s17=global
  wires:
  Battery/1 -> Bus Selector/1
  [c17] -> Breaker3/1, Breaker/1
  Bus Selector/2 -> Scope/2  "<Current (A)>"
  [d17] -> Breaker1/1, Breaker2/1
  Bus Selector/3 -> Scope/3  "<Voltage (V)>"
  Bus Selector/1 -> [s17], Scope/1  "<SOC (%)>"
  connections:
  Breaker2/LConn1 -- Breaker3/RConn1 -- Battery/LConn2
  Breaker1/LConn1 -- Battery/LConn1 -- Breaker/RConn1
  +/RConn1 -- Breaker/LConn1
  Series RLC Branch/LConn1 -- Breaker2/RConn1
  Series RLC Branch/RConn1 -- Breaker1/RConn1
  -/RConn1 -- Breaker3/LConn1

== system aa_IOT/Subsystem11/Subsystem13 ==
  Battery : spsBatteryLib/Battery  BatType=Lithium-Ion  NomV=12  NomQ=10  SOC=95  Batt_Tr=30  PresetModel=on  MaxQ=10  MinV=9  FullV=13.9678  Dis_rate=4.3478  R=0.012  Normal_OP=9.0435  expZone="[12.9646     0.491304]"
  Breaker{,1..3} (4 alike) : spsBreakerLib/Breaker  InitialState=0  SwitchingTimes="[1/60  5/60]"  External=on  BreakerResistance=0.01  SnubberResistance=1e6  SnubberCapacitance=inf  Measurements=None  MoreParameters=on  NoBreakLoop=off
  Bus Selector : BusSelector  OutputSignals=SOC (%),Current (A),Voltage (V)
  Display : Display
  MATLAB Function : MATLAB Function  TreatAsAtomicUnit=on
  Scope : Scope  NumInputPorts=3
  Series RLC Branch : spsSeriesRLCBranchLib/Series RLC Branch  LConnTagsString=__new0  RConnTagsString=__new0  BranchType=R  Resistance=1  Inductance=1e-3  SetiL0=off  InitialCurrent=0  Capacitance=1e-6  Setx0=off  InitialVoltage=0  Measurements=None
  + : PMIOPort  Side=Right
  - : PMIOPort  Port=2  Side=Right
  tag scope: s144=global
  wires:
  Battery/1 -> Bus Selector/1
  [s144] -> Breaker3/1, Breaker/1
  Bus Selector/2 -> MATLAB Function/3(Current), Scope/2  "<Current (A)>"
  [d14] -> Breaker1/1, Breaker2/1
  Bus Selector/3 -> MATLAB Function/2(Voltage), Scope/3  "<Voltage (V)>"
  Bus Selector/1 -> [s144], MATLAB Function/1(SOC), Scope/1  "<SOC (%)>"
  MATLAB Function/1(output) -> Display/1
  connections:
  Breaker2/LConn1 -- Breaker3/RConn1 -- Battery/LConn2
  Breaker1/LConn1 -- Battery/LConn1 -- Breaker/RConn1
  +/RConn1 -- Breaker/LConn1
  Series RLC Branch/LConn1 -- Breaker2/RConn1
  Series RLC Branch/RConn1 -- Breaker1/RConn1
  -/RConn1 -- Breaker3/LConn1

== system aa_IOT/Subsystem11/Subsystem14 ==
  Battery : spsBatteryLib/Battery  BatType=Lithium-Ion  NomV=12  NomQ=10  SOC=95  Batt_Tr=30  PresetModel=on  MaxQ=10  MinV=9  FullV=13.9678  Dis_rate=4.3478  R=0.012  Normal_OP=9.0435  expZone="[12.9646     0.491304]"
  Breaker{,1..3} (4 alike) : spsBreakerLib/Breaker  InitialState=0  SwitchingTimes="[1/60  5/60]"  External=on  BreakerResistance=0.01  SnubberResistance=1e6  SnubberCapacitance=inf  Measurements=None  MoreParameters=on  NoBreakLoop=off
  Bus Selector : BusSelector  OutputSignals=SOC (%),Current (A),Voltage (V)
  Scope : Scope  NumInputPorts=3
  Series RLC Branch : spsSeriesRLCBranchLib/Series RLC Branch  LConnTagsString=__new0  RConnTagsString=__new0  BranchType=R  Resistance=1  Inductance=1e-3  SetiL0=off  InitialCurrent=0  Capacitance=1e-6  Setx0=off  InitialVoltage=0  Measurements=None
  + : PMIOPort  Side=Right
  - : PMIOPort  Port=2  Side=Right
  tag scope: s1444=global
  wires:
  Battery/1 -> Bus Selector/1
  [c14] -> Breaker3/1, Breaker/1
  Bus Selector/2 -> Scope/2  "<Current (A)>"
  [d14] -> Breaker1/1, Breaker2/1
  Bus Selector/3 -> Scope/3  "<Voltage (V)>"
  Bus Selector/1 -> [s1444], Scope/1  "<SOC (%)>"
  connections:
  Breaker2/LConn1 -- Breaker3/RConn1 -- Battery/LConn2
  Breaker1/LConn1 -- Battery/LConn1 -- Breaker/RConn1
  +/RConn1 -- Breaker/LConn1
  Series RLC Branch/LConn1 -- Breaker2/RConn1
  Series RLC Branch/RConn1 -- Breaker1/RConn1
  -/RConn1 -- Breaker3/LConn1

== system aa_IOT/Subsystem11/Subsystem15 ==
  Battery : spsBatteryLib/Battery  BatType=Lithium-Ion  NomV=12  NomQ=10  SOC=95  Batt_Tr=30  PresetModel=on  MaxQ=10  MinV=9  FullV=13.9678  Dis_rate=4.3478  R=0.012  Normal_OP=9.0435  expZone="[12.9646     0.491304]"
  Breaker{,1..3} (4 alike) : spsBreakerLib/Breaker  InitialState=0  SwitchingTimes="[1/60  5/60]"  External=on  BreakerResistance=0.01  SnubberResistance=1e6  SnubberCapacitance=inf  Measurements=None  MoreParameters=on  NoBreakLoop=off
  Bus Selector : BusSelector  OutputSignals=SOC (%),Current (A),Voltage (V)
  Display : Display
  MATLAB Function : MATLAB Function  TreatAsAtomicUnit=on
  Scope : Scope  NumInputPorts=3
  Series RLC Branch : spsSeriesRLCBranchLib/Series RLC Branch  LConnTagsString=__new0  RConnTagsString=__new0  BranchType=R  Resistance=1  Inductance=1e-3  SetiL0=off  InitialCurrent=0  Capacitance=1e-6  Setx0=off  InitialVoltage=0  Measurements=None
  + : PMIOPort  Side=Right
  - : PMIOPort  Port=2  Side=Right
  tag scope: s12=global
  wires:
  Battery/1 -> Bus Selector/1
  [c12] -> Breaker3/1, Breaker/1
  Bus Selector/2 -> Scope/2, MATLAB Function/3(Current)  "<Current (A)>"
  [d12] -> Breaker1/1, Breaker2/1
  Bus Selector/3 -> MATLAB Function/2(Voltage), Scope/3  "<Voltage (V)>"
  Bus Selector/1 -> [s12], MATLAB Function/1(SOC), Scope/1  "<SOC (%)>"
  MATLAB Function/1(output) -> Display/1
  connections:
  Breaker2/LConn1 -- Breaker3/RConn1 -- Battery/LConn2
  Breaker1/LConn1 -- Battery/LConn1 -- Breaker/RConn1
  +/RConn1 -- Breaker/LConn1
  Series RLC Branch/LConn1 -- Breaker2/RConn1
  Series RLC Branch/RConn1 -- Breaker1/RConn1
  -/RConn1 -- Breaker3/LConn1

== system aa_IOT/Subsystem11/Subsystem16 ==
  Battery : spsBatteryLib/Battery  BatType=Lithium-Ion  NomV=12  NomQ=10  SOC=95  Batt_Tr=30  PresetModel=on  MaxQ=10  MinV=9  FullV=13.9678  Dis_rate=4.3478  R=0.012  Normal_OP=9.0435  expZone="[12.9646     0.491304]"
  Breaker{,1..3} (4 alike) : spsBreakerLib/Breaker  InitialState=0  SwitchingTimes="[1/60  5/60]"  External=on  BreakerResistance=0.01  SnubberResistance=1e6  SnubberCapacitance=inf  Measurements=None  MoreParameters=on  NoBreakLoop=off
  Bus Selector : BusSelector  OutputSignals=SOC (%),Current (A),Voltage (V)
  Scope : Scope  NumInputPorts=3
  Series RLC Branch : spsSeriesRLCBranchLib/Series RLC Branch  LConnTagsString=__new0  RConnTagsString=__new0  BranchType=R  Resistance=1  Inductance=1e-3  SetiL0=off  InitialCurrent=0  Capacitance=1e-6  Setx0=off  InitialVoltage=0  Measurements=None
  + : PMIOPort  Side=Right
  - : PMIOPort  Port=2  Side=Right
  tag scope: s25=global
  wires:
  Battery/1 -> Bus Selector/1
  [c25] -> Breaker3/1, Breaker/1
  Bus Selector/2 -> Scope/2  "<Current (A)>"
  [d25] -> Breaker1/1, Breaker2/1
  Bus Selector/3 -> Scope/3  "<Voltage (V)>"
  Bus Selector/1 -> [s25], Scope/1  "<SOC (%)>"
  connections:
  Breaker2/LConn1 -- Breaker3/RConn1 -- Battery/LConn2
  Breaker1/LConn1 -- Battery/LConn1 -- Breaker/RConn1
  +/RConn1 -- Breaker/LConn1
  Series RLC Branch/LConn1 -- Breaker2/RConn1
  Series RLC Branch/RConn1 -- Breaker1/RConn1
  -/RConn1 -- Breaker3/LConn1

== system aa_IOT/Subsystem11/Subsystem17 ==
  Battery : spsBatteryLib/Battery  BatType=Lithium-Ion  NomV=12  NomQ=10  SOC=95  Batt_Tr=30  PresetModel=on  MaxQ=10  MinV=9  FullV=13.9678  Dis_rate=4.3478  R=0.012  Normal_OP=9.0435  expZone="[12.9646     0.491304]"
  Breaker{,1..3} (4 alike) : spsBreakerLib/Breaker  InitialState=0  SwitchingTimes="[1/60  5/60]"  External=on  BreakerResistance=0.01  SnubberResistance=1e6  SnubberCapacitance=inf  Measurements=None  MoreParameters=on  NoBreakLoop=off
  Bus Selector : BusSelector  OutputSignals=SOC (%),Current (A),Voltage (V)
  Scope : Scope  NumInputPorts=3
  Series RLC Branch : spsSeriesRLCBranchLib/Series RLC Branch  LConnTagsString=__new0  RConnTagsString=__new0  BranchType=R  Resistance=1  Inductance=1e-3  SetiL0=off  InitialCurrent=0  Capacitance=1e-6  Setx0=off  InitialVoltage=0  Measurements=None
  + : PMIOPort  Side=Right
  - : PMIOPort  Port=2  Side=Right
  tag scope: s21=global
  wires:
  Battery/1 -> Bus Selector/1
  [c21] -> Breaker3/1, Breaker/1
  Bus Selector/2 -> Scope/2  "<Current (A)>"
  [d21] -> Breaker1/1, Breaker2/1
  Bus Selector/3 -> Scope/3  "<Voltage (V)>"
  Bus Selector/1 -> [s21], Scope/1  "<SOC (%)>"
  connections:
  Breaker2/LConn1 -- Breaker3/RConn1 -- Battery/LConn2
  Breaker1/LConn1 -- Battery/LConn1 -- Breaker/RConn1
  +/RConn1 -- Breaker/LConn1
  Series RLC Branch/LConn1 -- Breaker2/RConn1
  Series RLC Branch/RConn1 -- Breaker1/RConn1
  -/RConn1 -- Breaker3/LConn1

== system aa_IOT/Subsystem11/Subsystem18 ==
  Battery : spsBatteryLib/Battery  BatType=Lithium-Ion  NomV=12  NomQ=10  SOC=95  Batt_Tr=30  PresetModel=on  MaxQ=10  MinV=9  FullV=13.9678  Dis_rate=4.3478  R=0.012  Normal_OP=9.0435  expZone="[12.9646     0.491304]"
  Breaker{,1..3} (4 alike) : spsBreakerLib/Breaker  InitialState=0  SwitchingTimes="[1/60  5/60]"  External=on  BreakerResistance=0.01  SnubberResistance=1e6  SnubberCapacitance=inf  Measurements=None  MoreParameters=on  NoBreakLoop=off
  Bus Selector : BusSelector  OutputSignals=SOC (%),Current (A),Voltage (V)
  Scope : Scope  NumInputPorts=3
  Series RLC Branch : spsSeriesRLCBranchLib/Series RLC Branch  LConnTagsString=__new0  RConnTagsString=__new0  BranchType=R  Resistance=1  Inductance=1e-3  SetiL0=off  InitialCurrent=0  Capacitance=1e-6  Setx0=off  InitialVoltage=0  Measurements=None
  + : PMIOPort  Side=Right
  - : PMIOPort  Port=2  Side=Right
  tag scope: s9=global
  wires:
  Battery/1 -> Bus Selector/1
  [c9] -> Breaker3/1, Breaker/1
  Bus Selector/2 -> Scope/2  "<Current (A)>"
  [d9] -> Breaker1/1, Breaker2/1
  Bus Selector/3 -> Scope/3  "<Voltage (V)>"
  Bus Selector/1 -> [s9], Scope/1  "<SOC (%)>"
  connections:
  Breaker2/LConn1 -- Breaker3/RConn1 -- Battery/LConn2
  Breaker1/LConn1 -- Battery/LConn1 -- Breaker/RConn1
  +/RConn1 -- Breaker/LConn1
  Series RLC Branch/LConn1 -- Breaker2/RConn1
  Series RLC Branch/RConn1 -- Breaker1/RConn1
  -/RConn1 -- Breaker3/LConn1

== system aa_IOT/Subsystem11/Subsystem19 ==
  Battery : spsBatteryLib/Battery  BatType=Lithium-Ion  NomV=12  NomQ=10  SOC=95  Batt_Tr=30  PresetModel=on  MaxQ=10  MinV=9  FullV=13.9678  Dis_rate=4.3478  R=0.012  Normal_OP=9.0435  expZone="[12.9646     0.491304]"
  Breaker{,1..3} (4 alike) : spsBreakerLib/Breaker  InitialState=0  SwitchingTimes="[1/60  5/60]"  External=on  BreakerResistance=0.01  SnubberResistance=1e6  SnubberCapacitance=inf  Measurements=None  MoreParameters=on  NoBreakLoop=off
  Bus Selector : BusSelector  OutputSignals=SOC (%),Current (A),Voltage (V)
  Display : Display
  MATLAB Function : MATLAB Function  TreatAsAtomicUnit=on
  Scope : Scope  NumInputPorts=3
  Series RLC Branch : spsSeriesRLCBranchLib/Series RLC Branch  LConnTagsString=__new0  RConnTagsString=__new0  BranchType=R  Resistance=1  Inductance=1e-3  SetiL0=off  InitialCurrent=0  Capacitance=1e-6  Setx0=off  InitialVoltage=0  Measurements=None
  + : PMIOPort  Side=Right
  - : PMIOPort  Port=2  Side=Right
  tag scope: s10=global
  wires:
  Battery/1 -> Bus Selector/1
  [c10] -> Breaker3/1, Breaker/1
  Bus Selector/2 -> Scope/2, MATLAB Function/3(Current)  "<Current (A)>"
  [d10] -> Breaker1/1, Breaker2/1
  Bus Selector/3 -> MATLAB Function/2(Voltage), Scope/3  "<Voltage (V)>"
  Bus Selector/1 -> [s10], MATLAB Function/1(SOC), Scope/1  "<SOC (%)>"
  MATLAB Function/1(output) -> Display/1
  connections:
  Breaker2/LConn1 -- Breaker3/RConn1 -- Battery/LConn2
  Breaker1/LConn1 -- Battery/LConn1 -- Breaker/RConn1
  +/RConn1 -- Breaker/LConn1
  Series RLC Branch/LConn1 -- Breaker2/RConn1
  Series RLC Branch/RConn1 -- Breaker1/RConn1
  -/RConn1 -- Breaker3/LConn1

== system aa_IOT/Subsystem11/Subsystem2 ==
  Battery : spsBatteryLib/Battery  BatType=Lithium-Ion  NomV=12  NomQ=10  SOC=95  Batt_Tr=30  PresetModel=on  MaxQ=10  MinV=9  FullV=13.9678  Dis_rate=4.3478  R=0.012  Normal_OP=9.0435  expZone="[12.9646     0.491304]"
  Breaker{,1..3} (4 alike) : spsBreakerLib/Breaker  InitialState=0  SwitchingTimes="[1/60  5/60]"  External=on  BreakerResistance=0.01  SnubberResistance=1e6  SnubberCapacitance=inf  Measurements=None  MoreParameters=on  NoBreakLoop=off
  Bus Selector : BusSelector  OutputSignals=SOC (%),Current (A),Voltage (V)
  Display : Display
  MATLAB Function : MATLAB Function  TreatAsAtomicUnit=on
  Scope : Scope  NumInputPorts=3
  Series RLC Branch : spsSeriesRLCBranchLib/Series RLC Branch  LConnTagsString=__new0  RConnTagsString=__new0  BranchType=R  Resistance=1  Inductance=1e-3  SetiL0=off  InitialCurrent=0  Capacitance=1e-6  Setx0=off  InitialVoltage=0  Measurements=None
  + : PMIOPort  Side=Right
  - : PMIOPort  Port=2  Side=Right
  tag scope: s6=global
  wires:
  Battery/1 -> Bus Selector/1
  [c6] -> Breaker3/1, Breaker/1
  Bus Selector/2 -> MATLAB Function/3(Current), Scope/2  "<Current (A)>"
  [d6] -> Breaker1/1, Breaker2/1
  Bus Selector/3 -> MATLAB Function/2(Voltage), Scope/3  "<Voltage (V)>"
  Bus Selector/1 -> [s6], Scope/1, MATLAB Function/1(SOC)  "<SOC (%)>"
  MATLAB Function/1(output) -> Display/1
  connections:
  Breaker2/LConn1 -- Breaker3/RConn1 -- Battery/LConn2
  Breaker1/LConn1 -- Battery/LConn1 -- Breaker/RConn1
  +/RConn1 -- Breaker/LConn1
  Series RLC Branch/LConn1 -- Breaker2/RConn1
  Series RLC Branch/RConn1 -- Breaker1/RConn1
  -/RConn1 -- Breaker3/LConn1

== system aa_IOT/Subsystem11/Subsystem20 ==
  Battery : spsBatteryLib/Battery  BatType=Lithium-Ion  NomV=12  NomQ=10  SOC=95  Batt_Tr=30  PresetModel=on  MaxQ=10  MinV=9  FullV=13.9678  Dis_rate=4.3478  R=0.012  Normal_OP=9.0435  expZone="[12.9646     0.491304]"
  Breaker{,1..3} (4 alike) : spsBreakerLib/Breaker  InitialState=0  SwitchingTimes="[1/60  5/60]"  External=on  BreakerResistance=0.01  SnubberResistance=1e6  SnubberCapacitance=inf  Measurements=None  MoreParameters=on  NoBreakLoop=off
  Bus Selector : BusSelector  OutputSignals=SOC (%),Current (A),Voltage (V)
  Display : Display
  MATLAB Function : MATLAB Function  TreatAsAtomicUnit=on
  Scope : Scope  NumInputPorts=3
  Series RLC Branch : spsSeriesRLCBranchLib/Series RLC Branch  LConnTagsString=__new0  RConnTagsString=__new0  BranchType=R  Resistance=1  Inductance=1e-3  SetiL0=off  InitialCurrent=0  Capacitance=1e-6  Setx0=off  InitialVoltage=0  Measurements=None
  + : PMIOPort  Side=Right
  - : PMIOPort  Port=2  Side=Right
  tag scope: s8=global
  wires:
  Battery/1 -> Bus Selector/1
  [c8] -> Breaker3/1, Breaker/1
  Bus Selector/2 -> MATLAB Function/3(Current), Scope/2  "<Current (A)>"
  [d8] -> Breaker1/1, Breaker2/1
  Bus Selector/3 -> MATLAB Function/2(Voltage), Scope/3  "<Voltage (V)>"
  Bus Selector/1 -> [s8], Scope/1, MATLAB Function/1(SOC)  "<SOC (%)>"
  MATLAB Function/1(output) -> Display/1
  connections:
  Breaker2/LConn1 -- Breaker3/RConn1 -- Battery/LConn2
  Breaker1/LConn1 -- Battery/LConn1 -- Breaker/RConn1
  +/RConn1 -- Breaker/LConn1
  Series RLC Branch/LConn1 -- Breaker2/RConn1
  Series RLC Branch/RConn1 -- Breaker1/RConn1
  -/RConn1 -- Breaker3/LConn1

== system aa_IOT/Subsystem11/Subsystem21 ==
  Battery : spsBatteryLib/Battery  BatType=Lithium-Ion  NomV=12  NomQ=10  SOC=95  Batt_Tr=30  PresetModel=on  MaxQ=10  MinV=9  FullV=13.9678  Dis_rate=4.3478  R=0.012  Normal_OP=9.0435  expZone="[12.9646     0.491304]"
  Breaker{,1..3} (4 alike) : spsBreakerLib/Breaker  InitialState=0  SwitchingTimes="[1/60  5/60]"  External=on  BreakerResistance=0.01  SnubberResistance=1e6  SnubberCapacitance=inf  Measurements=None  MoreParameters=on  NoBreakLoop=off
  Bus Selector : BusSelector  OutputSignals=SOC (%),Current (A),Voltage (V)
  Scope : Scope  NumInputPorts=3
  Series RLC Branch : spsSeriesRLCBranchLib/Series RLC Branch  LConnTagsString=__new0  RConnTagsString=__new0  BranchType=R  Resistance=1  Inductance=1e-3  SetiL0=off  InitialCurrent=0  Capacitance=1e-6  Setx0=off  InitialVoltage=0  Measurements=None
  + : PMIOPort  Side=Right
  - : PMIOPort  Port=2  Side=Right
  tag scope: s7=global
  wires:
  Battery/1 -> Bus Selector/1
  [c7] -> Breaker3/1, Breaker/1
  Bus Selector/2 -> Scope/2  "<Current (A)>"
  [d7] -> Breaker1/1, Breaker2/1
  Bus Selector/3 -> Scope/3  "<Voltage (V)>"
  Bus Selector/1 -> [s7], Scope/1  "<SOC (%)>"
  connections:
  Breaker2/LConn1 -- Breaker3/RConn1 -- Battery/LConn2
  Breaker1/LConn1 -- Battery/LConn1 -- Breaker/RConn1
  +/RConn1 -- Breaker/LConn1
  Series RLC Branch/LConn1 -- Breaker2/RConn1
  Series RLC Branch/RConn1 -- Breaker1/RConn1
  -/RConn1 -- Breaker3/LConn1

== system aa_IOT/Subsystem11/Subsystem22 ==
  Battery : spsBatteryLib/Battery  BatType=Lithium-Ion  NomV=12  NomQ=10  SOC=95  Batt_Tr=30  PresetModel=on  MaxQ=10  MinV=9  FullV=13.9678  Dis_rate=4.3478  R=0.012  Normal_OP=9.0435  expZone="[12.9646     0.491304]"
  Breaker{,1..3} (4 alike) : spsBreakerLib/Breaker  InitialState=0  SwitchingTimes="[1/60  5/60]"  External=on  BreakerResistance=0.01  SnubberResistance=1e6  SnubberCapacitance=inf  Measurements=None  MoreParameters=on  NoBreakLoop=off
  Bus Selector : BusSelector  OutputSignals=SOC (%),Current (A),Voltage (V)
  Scope : Scope  NumInputPorts=3
  Series RLC Branch : spsSeriesRLCBranchLib/Series RLC Branch  LConnTagsString=__new0  RConnTagsString=__new0  BranchType=R  Resistance=1  Inductance=1e-3  SetiL0=off  InitialCurrent=0  Capacitance=1e-6  Setx0=off  InitialVoltage=0  Measurements=None
  + : PMIOPort  Side=Right
  - : PMIOPort  Port=2  Side=Right
  tag scope: s29=global
  wires:
  Battery/1 -> Bus Selector/1
  [c29] -> Breaker3/1, Breaker/1
  Bus Selector/2 -> Scope/2  "<Current (A)>"
  [d29] -> Breaker1/1, Breaker2/1
  Bus Selector/3 -> Scope/3  "<Voltage (V)>"
  Bus Selector/1 -> [s29], Scope/1  "<SOC (%)>"
  connections:
  Breaker2/LConn1 -- Breaker3/RConn1 -- Battery/LConn2
  Breaker1/LConn1 -- Battery/LConn1 -- Breaker/RConn1
  +/RConn1 -- Breaker/LConn1
  Series RLC Branch/LConn1 -- Breaker2/RConn1
  Series RLC Branch/RConn1 -- Breaker1/RConn1
  -/RConn1 -- Breaker3/LConn1

== system aa_IOT/Subsystem11/Subsystem23 ==
  Battery : spsBatteryLib/Battery  BatType=Lithium-Ion  NomV=12  NomQ=10  SOC=95  Batt_Tr=30  PresetModel=on  MaxQ=10  MinV=9  FullV=13.9678  Dis_rate=4.3478  R=0.012  Normal_OP=9.0435  expZone="[12.9646     0.491304]"
  Breaker{,1..3} (4 alike) : spsBreakerLib/Breaker  InitialState=0  SwitchingTimes="[1/60  5/60]"  External=on  BreakerResistance=0.01  SnubberResistance=1e6  SnubberCapacitance=inf  Measurements=None  MoreParameters=on  NoBreakLoop=off
  Bus Selector : BusSelector  OutputSignals=SOC (%),Current (A),Voltage (V)
  Display : Display
  MATLAB Function : MATLAB Function  TreatAsAtomicUnit=on
  Scope : Scope  NumInputPorts=3
  Series RLC Branch : spsSeriesRLCBranchLib/Series RLC Branch  LConnTagsString=__new0  RConnTagsString=__new0  BranchType=R  Resistance=1  Inductance=1e-3  SetiL0=off  InitialCurrent=0  Capacitance=1e-6  Setx0=off  InitialVoltage=0  Measurements=None
  + : PMIOPort  Side=Right
  - : PMIOPort  Port=2  Side=Right
  tag scope: s30=global
  wires:
  Battery/1 -> Bus Selector/1
  [c30] -> Breaker3/1, Breaker/1
  Bus Selector/2 -> MATLAB Function/3(Current), Scope/2  "<Current (A)>"
  [d30] -> Breaker1/1, Breaker2/1
  Bus Selector/3 -> MATLAB Function/2(Voltage), Scope/3  "<Voltage (V)>"
  Bus Selector/1 -> [s30], Scope/1, MATLAB Function/1(SOC)  "<SOC (%)>"
  MATLAB Function/1(output) -> Display/1
  connections:
  Breaker2/LConn1 -- Breaker3/RConn1 -- Battery/LConn2
  Breaker1/LConn1 -- Battery/LConn1 -- Breaker/RConn1
  +/RConn1 -- Breaker/LConn1
  Series RLC Branch/LConn1 -- Breaker2/RConn1
  Series RLC Branch/RConn1 -- Breaker1/RConn1
  -/RConn1 -- Breaker3/LConn1

== system aa_IOT/Subsystem11/Subsystem24 ==
  Battery : spsBatteryLib/Battery  BatType=Lithium-Ion  NomV=12  NomQ=10  SOC=95  Batt_Tr=30  PresetModel=on  MaxQ=10  MinV=9  FullV=13.9678  Dis_rate=4.3478  R=0.012  Normal_OP=9.0435  expZone="[12.9646     0.491304]"
  Breaker{,1..3} (4 alike) : spsBreakerLib/Breaker  InitialState=0  SwitchingTimes="[1/60  5/60]"  External=on  BreakerResistance=0.01  SnubberResistance=1e6  SnubberCapacitance=inf  Measurements=None  MoreParameters=on  NoBreakLoop=off
  Bus Selector : BusSelector  OutputSignals=SOC (%),Current (A),Voltage (V)
  Display : Display
  MATLAB Function : MATLAB Function  TreatAsAtomicUnit=on
  Scope : Scope  NumInputPorts=3
  Series RLC Branch : spsSeriesRLCBranchLib/Series RLC Branch  LConnTagsString=__new0  RConnTagsString=__new0  BranchType=R  Resistance=1  Inductance=1e-3  SetiL0=off  InitialCurrent=0  Capacitance=1e-6  Setx0=off  InitialVoltage=0  Measurements=None
  + : PMIOPort  Side=Right
  - : PMIOPort  Port=2  Side=Right
  tag scope: s26=global
  wires:
  Battery/1 -> Bus Selector/1
  [c26] -> Breaker3/1, Breaker/1
  Bus Selector/2 -> Scope/2, MATLAB Function/3(Current)  "<Current (A)>"
  [d26] -> Breaker1/1, Breaker2/1
  Bus Selector/3 -> MATLAB Function/2(Voltage), Scope/3  "<Voltage (V)>"
  Bus Selector/1 -> [s26], MATLAB Function/1(SOC), Scope/1  "<SOC (%)>"
  MATLAB Function/1(output) -> Display/1
  connections:
  Breaker2/LConn1 -- Breaker3/RConn1 -- Battery/LConn2
  Breaker1/LConn1 -- Battery/LConn1 -- Breaker/RConn1
  +/RConn1 -- Breaker/LConn1
  Series RLC Branch/LConn1 -- Breaker2/RConn1
  Series RLC Branch/RConn1 -- Breaker1/RConn1
  -/RConn1 -- Breaker3/LConn1

== system aa_IOT/Subsystem11/Subsystem25 ==
  Battery : spsBatteryLib/Battery  BatType=Lithium-Ion  NomV=12  NomQ=10  SOC=95  Batt_Tr=30  PresetModel=on  MaxQ=10  MinV=9  FullV=13.9678  Dis_rate=4.3478  R=0.012  Normal_OP=9.0435  expZone="[12.9646     0.491304]"
  Breaker{,1..3} (4 alike) : spsBreakerLib/Breaker  InitialState=0  SwitchingTimes="[1/60  5/60]"  External=on  BreakerResistance=0.01  SnubberResistance=1e6  SnubberCapacitance=inf  Measurements=None  MoreParameters=on  NoBreakLoop=off
  Bus Selector : BusSelector  OutputSignals=SOC (%),Current (A),Voltage (V)
  Display : Display
  MATLAB Function : MATLAB Function  TreatAsAtomicUnit=on
  Scope : Scope  NumInputPorts=3
  Series RLC Branch : spsSeriesRLCBranchLib/Series RLC Branch  LConnTagsString=__new0  RConnTagsString=__new0  BranchType=R  Resistance=1  Inductance=1e-3  SetiL0=off  InitialCurrent=0  Capacitance=1e-6  Setx0=off  InitialVoltage=0  Measurements=None
  + : PMIOPort  Side=Right
  - : PMIOPort  Port=2  Side=Right
  tag scope: s28=global
  wires:
  Battery/1 -> Bus Selector/1
  [c28] -> Breaker3/1, Breaker/1
  Bus Selector/2 -> MATLAB Function/3(Current), Scope/2  "<Current (A)>"
  [d28] -> Breaker1/1, Breaker2/1
  Bus Selector/3 -> MATLAB Function/2(Voltage), Scope/3  "<Voltage (V)>"
  Bus Selector/1 -> [s28], Scope/1, MATLAB Function/1(SOC)  "<SOC (%)>"
  MATLAB Function/1(output) -> Display/1
  connections:
  Breaker2/LConn1 -- Breaker3/RConn1 -- Battery/LConn2
  Breaker1/LConn1 -- Battery/LConn1 -- Breaker/RConn1
  +/RConn1 -- Breaker/LConn1
  Series RLC Branch/LConn1 -- Breaker2/RConn1
  Series RLC Branch/RConn1 -- Breaker1/RConn1
  -/RConn1 -- Breaker3/LConn1
